simulink model "Critically_Damped_SMD_System__1_ "  (R2024a)
settings: Solver=VariableStepAuto  StartTime=0.0  StopTime=10  RelTol=1e-3
settings Model: Creator=91839
settings SolverCC: AlgebraicLoopSolver=TrustRegion
settings DataIOCC: ExternalInput=data  LoadExternalInput=on  SaveFormat=Array  DSMLogging=off  ReturnWorkspaceOutputs=off
settings DebuggingCC: UnconnectedInputMsg=warning  UnconnectedOutputMsg=warning  UnconnectedLineMsg=warning
settings ModelReferenceCC: EnableRefExpFcnMdlSchedulingChecks=on
settings SFSimCC: CustomCodeUndefinedFunction=UseInterfaceOnly
settings RTWCC: GPUComputeCapability=3.5

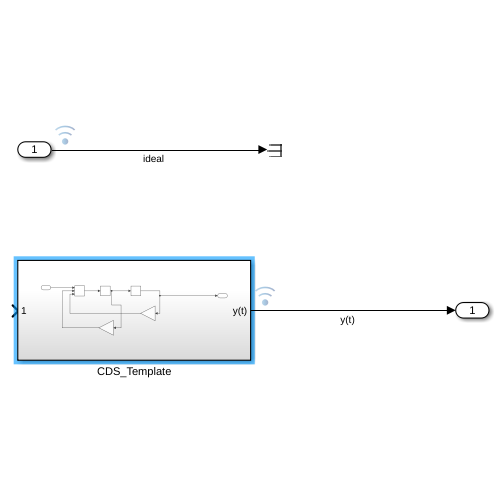
[thumbnail: Simulink's stored preview of the top-level diagram]
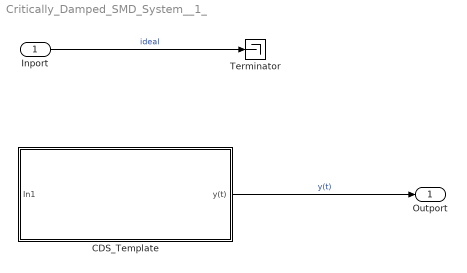
== system Critically_Damped_SMD_System__1_  ==
  Inport : Inport
  CDS_Template : Subsystem
  Terminator : Terminator
  Outport : Outport
  wires:
  Inport/1 -> Terminator/1  "ideal"
  CDS_Template/1(y(t)) -> Outport/1  "y(t)"

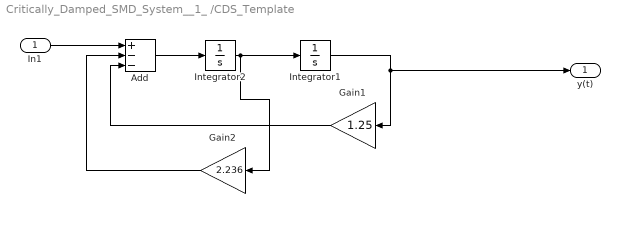
== system Critically_Damped_SMD_System__1_ /CDS_Template ==
  In1 : Inport
  Add : Sum  Inputs=+--
  Gain1 : Gain  Gain=1.25
  Gain2 : Gain  Gain=2.236
  Integrator1 : Integrator
  Integrator2 : Integrator
  y(t) : Outport
  wires:
  Add/1 -> Integrator2/1
  Integrator2/1 -> Gain2/1, Integrator1/1
  Integrator1/1 -> y(t)/1, Gain1/1
  Gain1/1 -> Add/3
  Gain2/1 -> Add/2
  In1/1 -> Add/1
